simulink model "controller_discrete"  (R2016a)
settings: Solver=FixedStepDiscrete  StartTime=0.0  StopTime=100  FixedStep=0.01  MaxStep=0.01  RelTol=1e-3
undefined symbols (not defined in the file): DiscIntNeverNeededParam, track_1
libraries: lflib x7
settings Model: Creator=The MathWorks, Inc.  LastModifiedBy=bures
settings SolverCC: ZeroCrossAlgorithm=Adaptive
settings DataIOCC: LimitDataPoints=on
settings DebuggingCC: AllowSymbolicDim=off
settings ModelReferenceCC: PropagateSignalLabelsOutOfModel=off
settings GRTTargetCC: GeneratePreprocessorConditionals=Use local settings

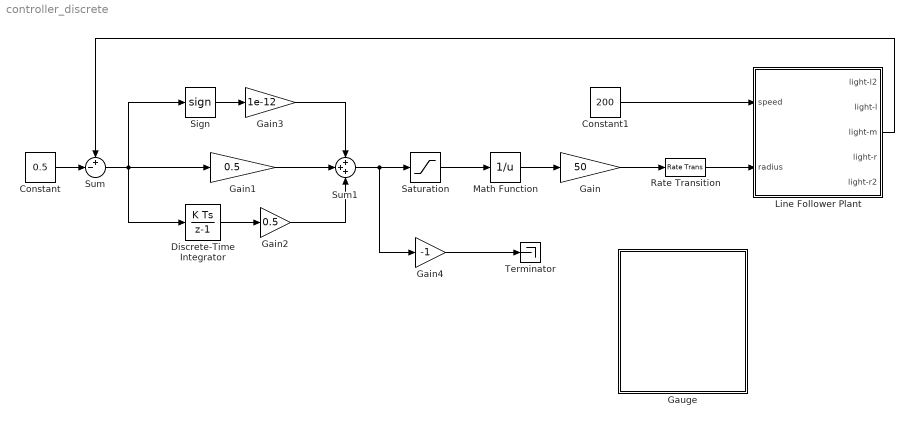
== system controller_discrete ==
  Constant : Constant  Value=0.5
  Constant1 : Constant  Value=200
  Discrete-Time Integrator : DiscreteIntegrator  InitialConditionSetting=State (most efficient)  SampleTime=-1  ICPrevOutput=DiscIntNeverNeededParam  ICPrevScaledInput=DiscIntNeverNeededParam
  Gain : Gain  Gain=50
  Gain1 : Gain  Gain=0.5
  Gain2 : Gain  Gain=0.5
  Gain3 : Gain  Gain=1e-12
  Gain4 : Gain  Gain=-1
  Gauge : Subsystem  DialogController=hmiCreateDDGDialog  IsWebBlock=on  mask(MWDashboardBlock){webBlockId=7db7642f-826f-4a11-a05c-208860c2e6f7, webBlockType=circulargauge, ShowInLibBrowser=on, ShowInitialText=on, HMISrcModelName=controller_discrete}
      mask prompts: webBlockId "WebBlock Id"; webBlockType "WebBlock Type"; HMISrcModelName "Source Model"
      mask Help: helpview([docroot '/mapfiles/simulink.map'], 'hmi_gauge')
      mask Display:
      | if strcmp(get_param(bdroot(gcb),'BlockDiagramType'), 'library')
      |     image([(matlabroot) '/toolbox/simulink/hmi/icons/CircularGauge.png']);
      | end
  Line Follower Plant : Subsystem  mask{initX=496, initY=1050, initAngle=3/2*pi, trackCData=track_1, trackSamplesPerM=1000}
      mask prompts: initX "X (in mm)"; initY "Y (in mm)"; initAngle "Angle (in rad)"; trackCData "Track map"; trackSamplesPerM "Track map samples/m"
  Math Function : Math  Operator=reciprocal  SaturateOnIntegerOverflow=on
  Rate Transition : RateTransition  OutPortSampleTime=0.01
  Saturation : Saturate  UpperLimit=50  LowerLimit=-50
  Sign : Signum
  Sum : Sum  Inputs=+-|
  Sum1 : Sum  Inputs=+++
  Terminator : Terminator
  wires:
  Constant1/1 -> Line Follower Plant/1(speed)
  Sum/1 -> Discrete-Time Integrator/1, Sign/1, Gain1/1
  Constant/1 -> Sum/2
  Line Follower Plant/3(light-m) -> Sum/1
  Math Function/1 -> Gain/1
  Sum1/1 -> Gain4/1, Saturation/1
  Discrete-Time Integrator/1 -> Gain2/1
  Saturation/1 -> Math Function/1
  Gain2/1 -> Sum1/3
  Gain1/1 -> Sum1/2
  Sign/1 -> Gain3/1
  Gain3/1 -> Sum1/1
  Gain/1 -> Rate Transition/1
  Rate Transition/1 -> Line Follower Plant/2(radius)
  Gain4/1 -> Terminator/1

== system controller_discrete/Gauge ==

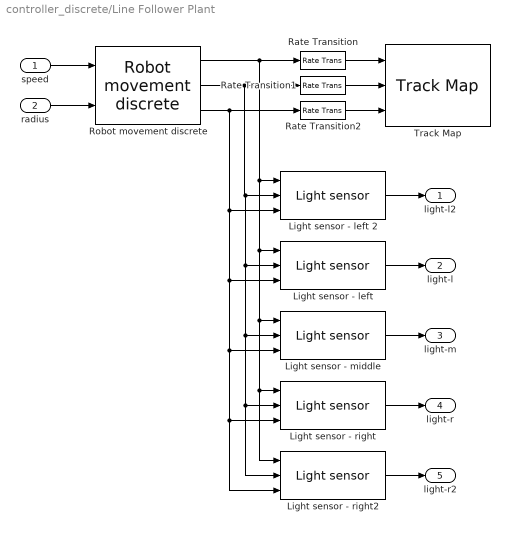
== system controller_discrete/Line Follower Plant ==
  speed : Inport
  radius : Inport  Port=2
  Light sensor - left : lflib/Light sensor  trackCData=trackCData  trackSamplesPerM=trackSamplesPerM  sensorPos=[150 30]
  Light sensor - left 2 : lflib/Light sensor  trackCData=trackCData  trackSamplesPerM=trackSamplesPerM  sensorPos=[150 70]
  Light sensor - middle : lflib/Light sensor  trackCData=trackCData  trackSamplesPerM=trackSamplesPerM  sensorPos=[150 0]
  Light sensor - right : lflib/Light sensor  trackCData=trackCData  trackSamplesPerM=trackSamplesPerM  sensorPos=[150 -30]
  Light sensor - right2 : lflib/Light sensor  trackCData=trackCData  trackSamplesPerM=trackSamplesPerM  sensorPos=[150 -70]
  Rate Transition : RateTransition
  Rate Transition1 : RateTransition
  Rate Transition2 : RateTransition
  Robot movement discrete : lflib/Robot movement discrete  initX=initX  initY=initY  initAngle=initAngle
  Track Map : lflib/Track Map  trackCData=trackCData  trackSamplesPerM=trackSamplesPerM
  light-l2 : Outport
  light-l : Outport  Port=2
  light-m : Outport  Port=3
  light-r : Outport  Port=4
  light-r2 : Outport  Port=5
  wires:
  Light sensor - right2/1 -> light-r2/1
  Light sensor - left/1 -> light-l/1
  Light sensor - middle/1 -> light-m/1
  Light sensor - left 2/1 -> light-l2/1
  Light sensor - right/1 -> light-r/1
  Robot movement discrete/1 -> Light sensor - right2/1, Light sensor - right/1, Light sensor - middle/1, Light sensor - left/1, Light sensor - left 2/1, Rate Transition/1
  Robot movement discrete/2 -> Light sensor - right2/2, Light sensor - right/2, Light sensor - middle/2, Light sensor - left/2, Light sensor - left 2/2, Rate Transition1/1
  radius/1 -> Robot movement discrete/2
  speed/1 -> Robot movement discrete/1
  Robot movement discrete/3 -> Light sensor - left/3, Light sensor - middle/3, Light sensor - right/3, Light sensor - right2/3, Light sensor - left 2/3, Rate Transition2/1
  Rate Transition/1 -> Track Map/1
  Rate Transition1/1 -> Track Map/2
  Rate Transition2/1 -> Track Map/3
